simulink model "discrete"  (R2020a)
settings: Solver=VariableStepAuto  StartTime=0.0  StopTime=100  RelTol=1e-3
libraries: discretizing x5
settings Model: Creator=user  LastModifiedBy=user

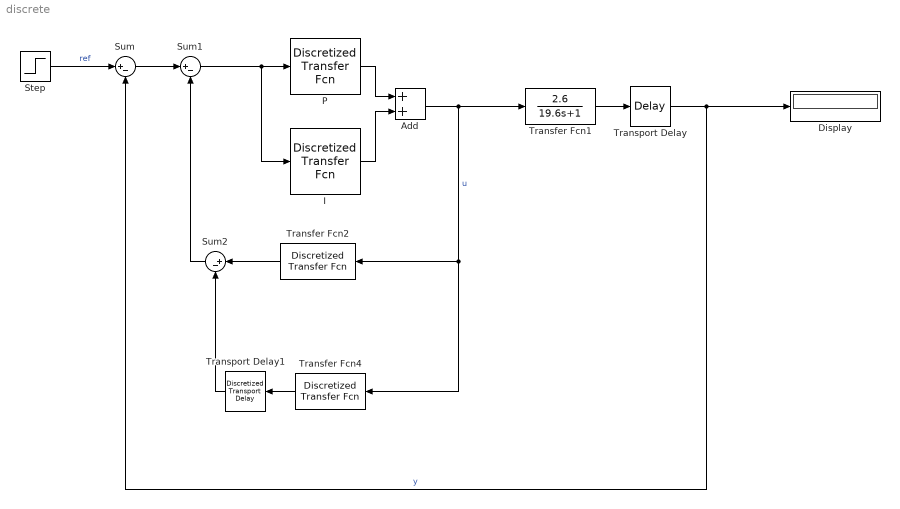
== system discrete ==
  Add : Sum
  Display : Display
  I : discretizing/Discretized Transfer Fcn  Numerator=[19.6/39]  Denominator=[19.6 0]  AbsTol=auto  SampleTime=2.5  method=tustin  Wc=1
      settings: SourceProductBaseCode=SL
  P : discretizing/Discretized Transfer Fcn  Numerator=[19.6/39]  Denominator=[0 1]  AbsTol=auto  SampleTime=2.5  method=tustin  Wc=1
      settings: SourceProductBaseCode=SL
  Step : Step  SampleTime=2.5  mask(DiscretizedSource){}
      mask init:
      | %tustin
  Sum : Sum  Inputs=|+-
  Sum1 : Sum  Inputs=|+-
  Sum2 : Sum  Inputs=|+-
  Transfer Fcn1 : TransferFcn  Numerator=[2.6]  Denominator=[19.6 1]
  Transfer Fcn2 : discretizing/Discretized Transfer Fcn  Numerator=[2.6]  Denominator=[19.6 1]  AbsTol=auto  SampleTime=2.5  method=tustin  Wc=1
      settings: SourceProductBaseCode=SL
  Transfer Fcn4 : discretizing/Discretized Transfer Fcn  Numerator=[2.6]  Denominator=[19.6 1]  AbsTol=auto  SampleTime=2.5  method=tustin  Wc=1
      settings: SourceProductBaseCode=SL
  Transport Delay : TransportDelay  DelayTime=5
  Transport Delay1 : discretizing/Discretized Transport Delay  delay=5  ic=0  SampleTime=2.5  rounding=Floor
      settings: SourceProductBaseCode=SL
  wires:
  I/1 -> Add/2
  Add/1 -> Transfer Fcn1/1, Transfer Fcn4/1, Transfer Fcn2/1  "u"
  Transfer Fcn2/1 -> Sum2/1
  Transfer Fcn4/1 -> Transport Delay1/1
  Transport Delay1/1 -> Sum2/2
  Sum1/1 -> I/1, P/1
  Sum/1 -> Sum1/1
  P/1 -> Add/1
  Sum2/1 -> Sum1/2
  Step/1 -> Sum/1  "ref"
  Transfer Fcn1/1 -> Transport Delay/1
  Transport Delay/1 -> Display/1, Sum/2  "y"
